simulink model "LC62_PIDControl_V6"  (R2022b)
settings: Solver=ode4  StartTime=0.0  StopTime=SimTime  FixedStep=1/500  RelTol=1e-3
model workspace (MAT data in the model file):
  Tr = 0.1
  freq = 0.002
  hover_w = 0.55
values from neighbouring files (symbols this model uses):
  b = 1.1    [initfun.m]
  c = 0.551    [initfun.m]
  Cll_beta = -0.0518    [initfun.m]
  Cll_del_A = -0.0369 * 5    (= -0.1845)    [initfun.m]
  Cll_del_R = 0.0026    [initfun.m]
  Cll_p = -0.4624    [initfun.m]
  Cll_r = 0.0218    [initfun.m]
  Cm_del_A = 0.001156    [initfun.m]
  Cm_del_E = -0.676    [initfun.m]
  Cn_beta = 0.0866    [initfun.m]
  Cn_del_A = -0.000385    [initfun.m]
  Cn_del_R = -0.0190    (= -0.019)    [initfun.m]
  Cn_p = -0.0048    [initfun.m]
  Cn_r = -0.0723    [initfun.m]
  Cy_beta = -1.1269    [initfun.m]
  Cy_del_R = 0.0534    [initfun.m]
  Cy_p = 0.0    (= 0)    [initfun.m]
  Cy_r = 0.2374    [initfun.m]
  d = 0.849    [initfun.m]
  dx1 = 0.9325+0.049    (= 0.9815)    [initfun.m]
  dx2 = 0.0725-0.049    (= 0.0235)    [initfun.m]
  dx3 = 1.1725-0.049    (= 1.1235)    [initfun.m]
  dy1 = 0.717 + temp_y    (= 0.717)    [initfun.m]
  dy2 = 0.717 - temp_y    (= 0.717)    [initfun.m]
  g = 9.81    [initfun.m]
  m = 41.97    [initfun.m]
  S = S1 + S2    (= 0.8522)    [initfun.m]
  S2 = 0.5898    [initfun.m]
undefined symbols (not defined in the file or in its folder): d2r, Earth, F, Light, MIL, sigbuilder_block, WGS84
libraries: simulink_extras x50, slpidlib x14, simulink x11, dspstat3 x5, aerolibwind2 x3, sharedTrackingLibrary x2, aerolibasang x2, aerolibtransform2 x2, robotcorelib x1, uavutilslib x1, uavalgslib x1, aerolibnav x1
(part 1 of 4)
settings Model: Creator=CNU_UASG  LastModifiedBy=박범준
settings DebuggingCC: UnconnectedInputMsg=warning  UnconnectedOutputMsg=warning  UnconnectedLineMsg=warning  UnderSpecifiedDimensionMsg=warning
settings ModelReferenceCC: EnableRefExpFcnMdlSchedulingChecks=on
settings RTWCC: DLArmComputeVersion=19.05

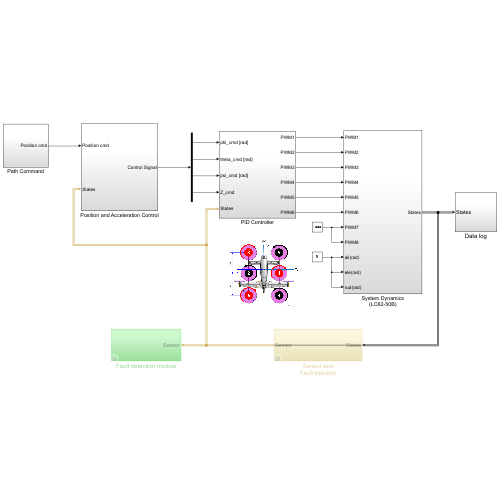
[thumbnail: Simulink's stored preview of the top-level diagram]
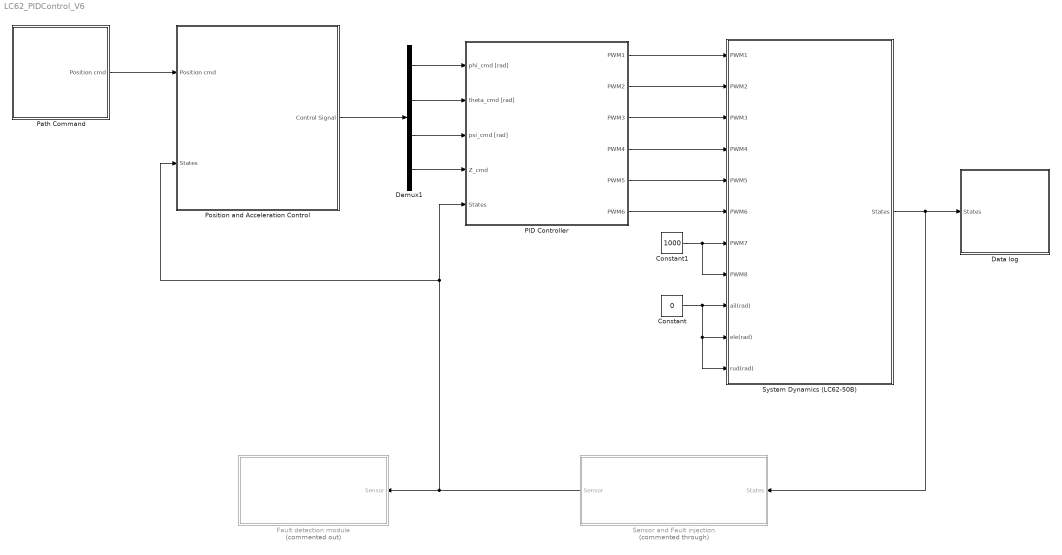
== system LC62_PIDControl_V6 ==
  Constant : Constant  Value=0
  Constant1 : Constant  Value=1000
  Data log : Subsystem
  Demux1 : Demux
  Fault detection module : Subsystem  Commented=on
  PID Controller : Subsystem
  Path Command : Subsystem
  Position and Acceleration Control : Subsystem
  Sensor and Fault injection : Subsystem  Commented=through
  System Dynamics (LC62-50B) : Subsystem
  wires:
  PID Controller/1(PWM1) -> System Dynamics (LC62-50B)/1(PWM1)
  PID Controller/2(PWM2) -> System Dynamics (LC62-50B)/2(PWM2)
  PID Controller/3(PWM3) -> System Dynamics (LC62-50B)/3(PWM3)
  PID Controller/4(PWM4) -> System Dynamics (LC62-50B)/4(PWM4)
  PID Controller/5(PWM5) -> System Dynamics (LC62-50B)/5(PWM5)
  PID Controller/6(PWM6) -> System Dynamics (LC62-50B)/6(PWM6)
  Constant1/1 -> System Dynamics (LC62-50B)/8(PWM8), System Dynamics (LC62-50B)/7(PWM7)
  Constant/1 -> System Dynamics (LC62-50B)/9(ail(rad)), System Dynamics (LC62-50B)/11(rud(rad)), System Dynamics (LC62-50B)/10(ele(rad))
  Demux1/2 -> PID Controller/2(theta_cmd [rad])
  Demux1/1 -> PID Controller/1(phi_cmd [rad])
  Demux1/3 -> PID Controller/3(psi_cmd [rad])
  Demux1/4 -> PID Controller/4(Z_cmd)
  System Dynamics (LC62-50B)/1(States) -> Sensor and Fault injection/1(States), Data log/1(States)
  Position and Acceleration Control/1(Control Signal) -> Demux1/1
  Path Command/1(Position cmd) -> Position and Acceleration Control/1(Position cmd)
  Sensor and Fault injection/1(Sensor) -> Fault detection module/1(Sensor), Position and Acceleration Control/2(States), PID Controller/5(States)

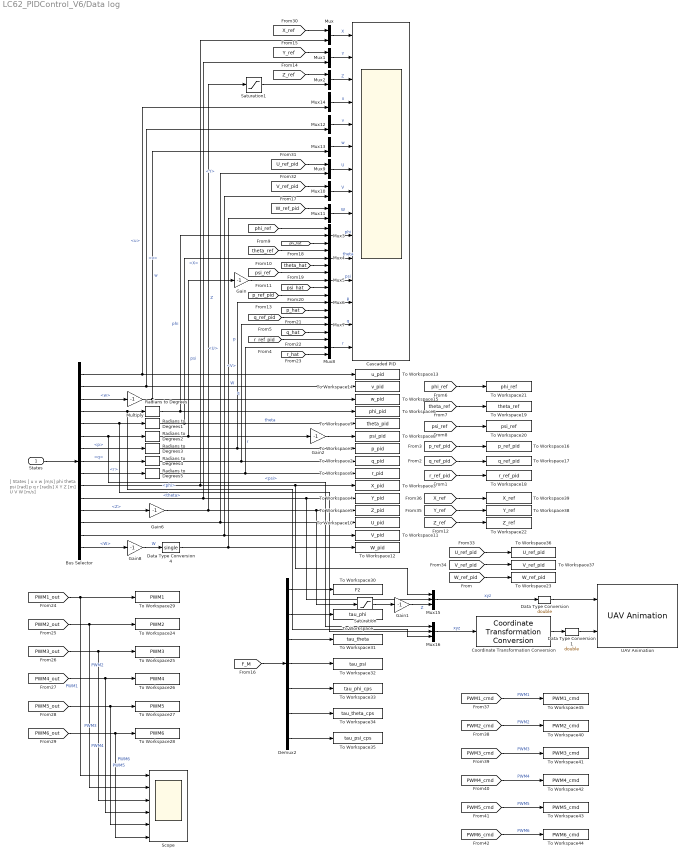
== system LC62_PIDControl_V6/Data log ==
  note: [ States ]
      | u v w [m/s]
      | phi theta psi [rad]
      | p q r [rad/s]
      | X Y Z [m]
      | U V W [m/s]
  States : Inport
  Bus Selector : BusSelector  OutputSignals=u,v,w,phi,theta,psi,p,q,r,X,Y,Z,U,V,W
  Cascaded PID : Scope  NumInputPorts=15
  Coordinate Transformation Conversion : robotcorelib/Coordinate Transformation Conversion  InputRepresentation=Euler Angles  InputEulerSequence=ZYX  ShowTrVecInputPort=on  OutputRepresentation=Quaternion  OutputEulerSequence=ZYX  ShowTrVecOutputPort=on  SimulateUsing=Code generation
  Data Type Conversion : DataTypeConversion  OutDataTypeStr=double  SaturateOnIntegerOverflow=off  RndMeth=Floor
  Data Type Conversion1 : DataTypeConversion  OutDataTypeStr=double  SaturateOnIntegerOverflow=off  RndMeth=Floor
  Data Type Conversion4 : DataTypeConversion  OutDataTypeStr=single  SaturateOnIntegerOverflow=off  RndMeth=Floor
  Demux2 : Demux  Outputs=7
  Gain{,1..2,6,8} (5 alike) : Gain  Gain=-1
  Multiply : Gain  Gain=-1
  Mux{,1..2,9..14} (9 alike) : Mux  Inputs=2
  Mux{3..8,15..16} (8 alike) : Mux  Inputs=3
  Radians to Degrees{,1..5} (6 alike) : simulink_extras/Transformations/Radians to Degrees
  Saturation : Saturate  UpperLimit=500  LowerLimit=0
  Saturation1 : Saturate  UpperLimit=500  LowerLimit=0
  Scope : Scope  NumInputPorts=6
  To Workspace : ToWorkspace  VariableName=tau_phi  SampleTime=-1
  To Workspace1 : ToWorkspace  VariableName=p_pid  SampleTime=-1
  To Workspace10 : ToWorkspace  VariableName=U_pid  SampleTime=-1
  To Workspace11 : ToWorkspace  VariableName=V_pid  SampleTime=-1
  To Workspace12 : ToWorkspace  VariableName=W_pid  SampleTime=-1
  To Workspace13 : ToWorkspace  VariableName=u_pid  SampleTime=-1
  To Workspace14 : ToWorkspace  VariableName=v_pid  SampleTime=-1
  To Workspace15 : ToWorkspace  VariableName=w_pid  SampleTime=-1
  To Workspace16 : ToWorkspace  VariableName=p_ref_pid  SampleTime=-1
  To Workspace17 : ToWorkspace  VariableName=q_ref_pid  SampleTime=-1
  To Workspace18 : ToWorkspace  VariableName=r_ref_pid  SampleTime=-1
  To Workspace19 : ToWorkspace  VariableName=theta_ref  SampleTime=-1
  To Workspace2 : ToWorkspace  VariableName=q_pid  SampleTime=-1
  To Workspace20 : ToWorkspace  VariableName=psi_ref  SampleTime=-1
  To Workspace21 : ToWorkspace  VariableName=phi_ref  SampleTime=-1
  To Workspace22 : ToWorkspace  VariableName=Z_ref  SampleTime=-1
  To Workspace23 : ToWorkspace  VariableName=W_ref_pid  SampleTime=-1
  To Workspace24 : ToWorkspace  VariableName=PWM2  SampleTime=-1
  To Workspace25 : ToWorkspace  VariableName=PWM3  SampleTime=-1
  To Workspace26 : ToWorkspace  VariableName=PWM4  SampleTime=-1
  To Workspace27 : ToWorkspace  VariableName=PWM5  SampleTime=-1
  To Workspace28 : ToWorkspace  VariableName=PWM6  SampleTime=-1
  To Workspace29 : ToWorkspace  VariableName=PWM1  SampleTime=-1
  To Workspace3 : ToWorkspace  VariableName=X_pid  SampleTime=-1
  To Workspace30 : ToWorkspace  VariableName=Fz  SampleTime=-1
  To Workspace31 : ToWorkspace  VariableName=tau_theta  SampleTime=-1
  To Workspace32 : ToWorkspace  VariableName=tau_psi  SampleTime=-1
  To Workspace33 : ToWorkspace  VariableName=tau_phi_cps  SampleTime=-1
  To Workspace34 : ToWorkspace  VariableName=tau_theta_cps  SampleTime=-1
  To Workspace35 : ToWorkspace  VariableName=tau_psi_cps  SampleTime=-1
  To Workspace36 : ToWorkspace  VariableName=U_ref_pid  SampleTime=-1
  To Workspace37 : ToWorkspace  VariableName=V_ref_pid  SampleTime=-1
  To Workspace38 : ToWorkspace  VariableName=Y_ref  SampleTime=-1
  To Workspace39 : ToWorkspace  VariableName=X_ref  SampleTime=-1
  To Workspace4 : ToWorkspace  VariableName=Y_pid  SampleTime=-1
  To Workspace40 : ToWorkspace  VariableName=PWM2_cmd  SampleTime=-1
  To Workspace41 : ToWorkspace  VariableName=PWM3_cmd  SampleTime=-1
  To Workspace42 : ToWorkspace  VariableName=PWM4_cmd  SampleTime=-1
  To Workspace43 : ToWorkspace  VariableName=PWM5_cmd  SampleTime=-1
  To Workspace44 : ToWorkspace  VariableName=PWM6_cmd  SampleTime=-1
  To Workspace45 : ToWorkspace  VariableName=PWM1_cmd  SampleTime=-1
  To Workspace5 : ToWorkspace  VariableName=Z_pid  SampleTime=-1
  To Workspace6 : ToWorkspace  VariableName=phi_pid  SampleTime=-1
  To Workspace7 : ToWorkspace  VariableName=theta_pid  SampleTime=-1
  To Workspace8 : ToWorkspace  VariableName=psi_pid  SampleTime=-1
  To Workspace9 : ToWorkspace  VariableName=r_pid  SampleTime=-1
  UAV Animation : uavutilslib/UAV Animation  UAVType=Multirotor  UAVSize=1  InertialZDirection=Down  SampleTime=1
  wires:
  Bus Selector/12 -> Gain6/1  "<Z>"
  Bus Selector/8 -> Radians to Degrees4/1  "<q>"
  Bus Selector/9 -> Radians to Degrees5/1  "<r>"
  Bus Selector/4 -> Mux16/3, Radians to Degrees/1  "<phi>"
  Bus Selector/5 -> Mux16/2, Radians to Degrees1/1  "<theta>"
  Bus Selector/7 -> Radians to Degrees3/1  "<p>"
  States/1 -> Bus Selector/1
  Bus Selector/15 -> Gain8/1  "<W>"
  Bus Selector/6 -> Mux16/1, Radians to Degrees2/1  "<psi>"
  Bus Selector/3 -> Multiply/1  "<w>"
  Bus Selector/10 -> Mux15/1, To Workspace3/1, Mux/2  "<X>"
  Bus Selector/11 -> Mux15/2, To Workspace4/1, Mux1/2  "<Y>"
  Gain6/1 -> Saturation/1, To Workspace5/1, Saturation1/1  "Z"
  Radians to Degrees3/1 -> To Workspace1/1, Mux6/2  "p"
  Radians to Degrees4/1 -> To Workspace2/1, Mux7/2  "q"
  Radians to Degrees5/1 -> To Workspace9/1, Mux8/2  "r"
  Gain8/1 -> Data Type Conversion4/1  "W"
  Bus Selector/14 -> To Workspace11/1, Mux10/2  "<V>"
  Bus Selector/13 -> To Workspace10/1, Mux9/2  "<U>"
  Radians to Degrees2/1 -> Gain2/1, Gain/1  "psi"
  Radians to Degrees1/1 -> To Workspace7/1, Mux4/2  "theta"
  Radians to Degrees/1 -> To Workspace6/1, Mux3/2  "phi"
  Multiply/1 -> To Workspace15/1, Mux13/2  "w"
  Bus Selector/2 -> To Workspace14/1, Mux12/2  "<v>"
  Bus Selector/1 -> Mux14/2, To Workspace13/1  "<u>"
  Mux2/1 -> Cascaded PID/3  "Z"
  Mux/1 -> Cascaded PID/1  "X"
  Mux1/1 -> Cascaded PID/2  "Y"
  Mux10/1 -> Cascaded PID/8  "V"
  Mux9/1 -> Cascaded PID/7  "U"
  Mux11/1 -> Cascaded PID/9  "W"
  Mux13/1 -> Cascaded PID/6  "w"
  Mux12/1 -> Cascaded PID/5  "v"
  [q_ref_pid] -> Mux7/1
  [p_ref_pid] -> Mux6/1
  [r_ref_pid] -> Mux8/1
  Mux3/1 -> Cascaded PID/10  "phi"
  Mux4/1 -> Cascaded PID/11  "theta"
  Mux5/1 -> Cascaded PID/12  "psi"
  Mux6/1 -> Cascaded PID/13  "p"
  Mux7/1 -> Cascaded PID/14  "q"
  Mux8/1 -> Cascaded PID/15  "r"
  [psi_ref] -> To Workspace20/1
  [phi_ref] -> To Workspace21/1
  [theta_ref] -> To Workspace19/1
  [phi_ref] -> Mux3/1
  [theta_ref] -> Mux4/1
  [psi_ref] -> Mux5/1
  [Z_ref] -> To Workspace22/1
  [Z_ref] -> Mux2/1
  [W_ref_pid] -> To Workspace23/1
  [p_ref_pid] -> To Workspace16/1
  [q_ref_pid] -> To Workspace17/1
  [r_ref_pid] -> To Workspace18/1
  [F_M] -> Demux2/1
  Demux2/5 -> To Workspace33/1
  Demux2/6 -> To Workspace34/1
  Demux2/7 -> To Workspace35/1
  Demux2/4 -> To Workspace32/1
  Demux2/3 -> To Workspace31/1
  Demux2/2 -> To Workspace/1
  Demux2/1 -> To Workspace30/1
  [W_ref_pid] -> Mux11/1
  [PWM1_out] -> Scope/1, To Workspace29/1  "PWM1"
  [PWM2_out] -> Scope/2, To Workspace24/1  "PWM2"
  [PWM3_out] -> Scope/3, To Workspace25/1  "PWM3"
  [PWM4_out] -> Scope/4, To Workspace26/1  "PWM4"
  [PWM5_out] -> Scope/5, To Workspace27/1  "PWM5"
  [PWM6_out] -> To Workspace28/1, Scope/6  "PWM6"
  [phi_hat] -> Mux3/3
  [theta_hat] -> Mux4/3
  [psi_hat] -> Mux5/3
  [p_hat] -> Mux6/3
  [q_hat] -> Mux7/3
  [r_hat] -> Mux8/3
  Coordinate Transformation Conversion/1 -> Data Type Conversion1/1
  Data Type Conversion/1 -> UAV Animation/1
  Mux15/1 -> Data Type Conversion/1  "xyz"
  Mux16/1 -> Coordinate Transformation Conversion/1  "xyz"
  Data Type Conversion4/1 -> To Workspace12/1, Mux11/2  "W"
  [Y_ref] -> Mux1/1
  [X_ref] -> Mux/1
  Data Type Conversion1/1 -> UAV Animation/2
  Gain1/1 -> Mux15/3  "Z"
  [U_ref_pid] -> Mux9/1
  [V_ref_pid] -> Mux10/1
  Mux14/1 -> Cascaded PID/4  "u"
  [U_ref_pid] -> To Workspace36/1
  [V_ref_pid] -> To Workspace37/1
  [Y_ref] -> To Workspace38/1
  [X_ref] -> To Workspace39/1
  [PWM6_cmd] -> To Workspace44/1  "PWM6"
  [PWM5_cmd] -> To Workspace43/1  "PWM5"
  [PWM4_cmd] -> To Workspace42/1  "PWM4"
  [PWM3_cmd] -> To Workspace41/1  "PWM3"
  [PWM2_cmd] -> To Workspace40/1  "PWM2"
  [PWM1_cmd] -> To Workspace45/1  "PWM1"
  Saturation/1 -> Gain1/1
  Saturation1/1 -> Mux2/2
  Gain/1 -> Mux5/2
  Gain2/1 -> To Workspace8/1

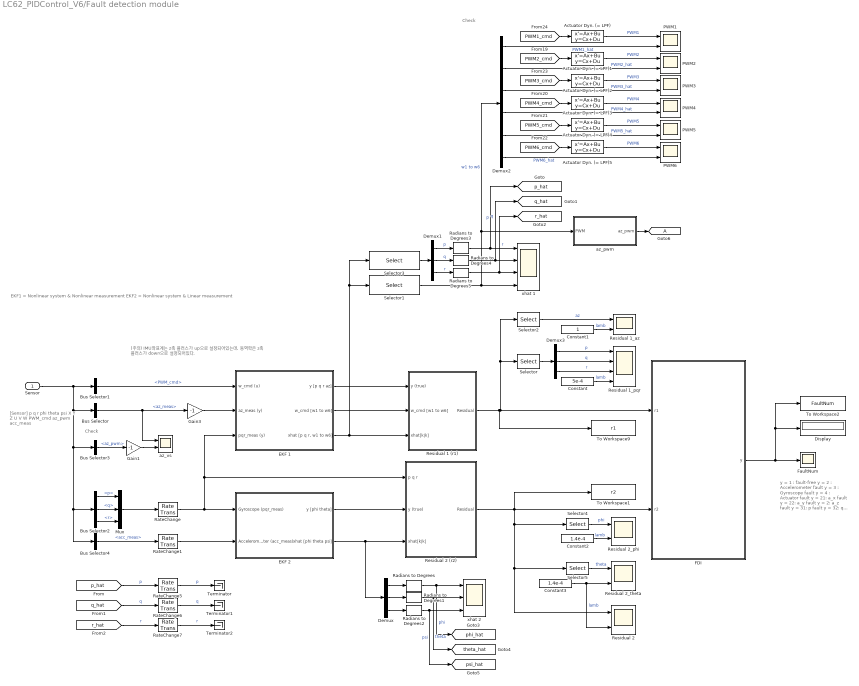
== system LC62_PIDControl_V6/Fault detection module ==
  note: (주의) IMU좌표계는 z축 플러스가 up으로 설정되어있는데,
      | 동역학은 z축 플러스가 down으로 설정되어있다.
  note: Check
  note: y = 1 : fault-free
      | y = 2 : Accelerometer fault
      | y = 3 : Gyroscope fault
      | y = 4 : Actuator fault
      |
      | y = 21: a_x fault
      | y = 22: a_y fault
      | y = 2: a_z fault
      |
      | y = 31: p fault
      | y = 32: q fault
      | y = 33: r fault
  note: EKF1 = Nonlinear system & Nonlinear measurement
      |
      | EKF2 = Nonlinear system & Linear measurement
  note: [Sensor]
      | p q r
      | phi theta psi
      | X Y Z
      | U V W
      | PWM_cmd
      | az_pwm
      | acc_meas
  note: Check
  Sensor : Inport
  Actuator Dyn. (= LPF){,1..5} (6 alike) : StateSpace  A=-1/Tr  B=1/Tr  D=0  InitialCondition=hover_w
  Bus Selector : BusSelector  OutputSignals=acc_meas.az_meas
  Bus Selector1 : BusSelector  OutputSignals=PWM_cmd
  Bus Selector2 : BusSelector  OutputSignals=p,q,r
  Bus Selector3 : BusSelector  OutputSignals=az_pwm
  Bus Selector4 : BusSelector  OutputSignals=acc_meas
  Constant : Constant  Value=5e-4
  Constant1 : Constant
  Constant2 : Constant  Value=1.4e-4
  Constant3 : Constant  Value=1.4e-4
  Demux : Demux  Outputs=3
  Demux1 : Demux  Outputs=3
  Demux2 : Demux  Outputs=6
  Demux3 : Demux  Outputs=3
  Display : Display
  EKF 1 : Subsystem
  EKF 2 : Subsystem
  FDI : MATLAB Function  TreatAsAtomicUnit=on
  FaultNum : Scope
  Gain1 : Gain  Gain=-1
  Gain3 : Gain  Gain=-1
  Goto6 : Goto  TagVisibility=global
  Mux : Mux  Inputs=3
  PWM{1..6} (6 alike) : Scope  NumInputPorts=2
  Radians to Degrees{,1..5} (6 alike) : simulink_extras/Transformations/Radians to Degrees
  RateChange : RateTransition  OutPortSampleTime=0.05
  RateChange1 : RateTransition  OutPortSampleTime=0.05
  RateChange5 : RateTransition  OutPortSampleTime=1/500
  RateChange6 : RateTransition  OutPortSampleTime=1/500
  RateChange7 : RateTransition  OutPortSampleTime=1/500
  Residual 1 (r1) : Subsystem
  Residual 1_az : Scope  NumInputPorts=2
  Residual 1_pqr : Scope  NumInputPorts=4
  Residual 2 : Scope  NumInputPorts=2
  Residual 2 (r2) : Subsystem
  Residual 2_phi : Scope  NumInputPorts=2
  Residual 2_theta : Scope  NumInputPorts=2
  Selector : Selector  InputPortWidth=4  IndexOptions=Index vector (dialog)  Indices=[1:3]  OutputSizes=1
  Selector1 : Selector  InputPortWidth=9  IndexOptions=Index vector (dialog)  Indices=[4:9]  OutputSizes=1
  Selector2 : Selector  InputPortWidth=4  IndexOptions=Index vector (dialog)  Indices=[4]  OutputSizes=1
  Selector3 : Selector  InputPortWidth=9  IndexOptions=Index vector (dialog)  Indices=[1:3]  OutputSizes=1
  Selector4 : Selector  InputPortWidth=2  IndexOptions=Index vector (dialog)  Indices=[1]  OutputSizes=1
  Selector5 : Selector  InputPortWidth=2  IndexOptions=Index vector (dialog)  Indices=[2]  OutputSizes=1
  Terminator : Terminator
  Terminator1 : Terminator
  Terminator2 : Terminator
  To Workspace1 : ToWorkspace  VariableName=r2  SampleTime=-1
  To Workspace2 : ToWorkspace  VariableName=FaultNum  SampleTime=-1
  To Workspace9 : ToWorkspace  VariableName=r1  SampleTime=-1
  az_pwm : MATLAB Function  TreatAsAtomicUnit=on
  az_vs : Scope  NumInputPorts=2
  xhat 1 : Scope  NumInputPorts=4
  xhat 2 : Scope  NumInputPorts=3
  tag scope: p_hat=global, phi_hat=global, psi_hat=global, q_hat=global, r_hat=global, theta_hat=global
  wires:
  Sensor/1 -> Bus Selector/1, Bus Selector3/1, Bus Selector4/1, Bus Selector2/1, Bus Selector1/1
  [q_hat] -> RateChange6/1  "q"
  Demux1/2 -> Radians to Degrees4/1  "q"
  EKF 1/2(w_cmd [w1 to w6]) -> Residual 1 (r1)/2(w_cmd [w1 to w6])
  Selector4/1 -> Residual 2_phi/1  "phi"
  Radians to Degrees2/1 -> xhat 2/3, [psi_hat]  "psi"
  Radians to Degrees5/1 -> [r_hat], xhat 1/3  "r"
  EKF 1/3("xhat [p q r, w1 to w6]") -> Residual 1 (r1)/3(xhat[k|k]), Selector3/1, Selector1/1
  EKF 1/1(y [p q r az]) -> Residual 1 (r1)/1(y (true))
  RateChange5/1 -> Terminator/1  "p"
  Demux1/3 -> Radians to Degrees5/1  "r"
  Demux/1 -> Radians to Degrees/1
  Radians to Degrees/1 -> xhat 2/1, [phi_hat]  "phi"
  EKF 2/1(y [phi theta]) -> Residual 2 (r2)/2(y (true))
  Radians to Degrees1/1 -> xhat 2/2, [theta_hat]  "theta"
  Gain3/1 -> EKF 1/2(az_meas (y))
  Bus Selector2/3 -> Mux/3  "<r>"
  Bus Selector4/1 -> RateChange1/1  "<acc_meas>"
  Bus Selector2/1 -> Mux/1  "<p>"
  FDI/1(y) -> To Workspace2/1, Display/1, FaultNum/1
  Demux1/1 -> Radians to Degrees3/1  "p"
  RateChange6/1 -> Terminator1/1  "q"
  Selector1/1 -> Demux2/1, az_pwm/1(PWM), xhat 1/4  "w1 to w6"
  Bus Selector/1 -> Gain3/1, az_vs/1  "<az_meas>"
  Selector3/1 -> Demux1/1
  [r_hat] -> RateChange7/1  "r"
  [p_hat] -> RateChange5/1  "p"
  EKF 2/2(xhat [phi theta psi]) -> Demux/1, Residual 2 (r2)/3(xhat[k|k])
  RateChange1/1 -> EKF 2/2(Accelerometer (acc_meas))
  Bus Selector2/2 -> Mux/2  "<q>"
  Bus Selector1/1 -> EKF 1/1(w_cmd (u))  "<PWM_cmd>"
  RateChange7/1 -> Terminator2/1  "r"
  Residual 1 (r1)/1(Residual) -> Selector/1, Selector2/1, FDI/1(r1), To Workspace9/1
  RateChange/1 -> Residual 2 (r2)/1(p q r), EKF 1/3(pqr_meas (y)), EKF 2/1(Gyroscope (pqr_meas))
  Demux/2 -> Radians to Degrees1/1
  Radians to Degrees3/1 -> [p_hat], xhat 1/1  "p"
  Residual 2 (r2)/1(Residual) -> Selector5/1, Residual 2/1, Selector4/1, FDI/2(r2), To Workspace1/1
  Mux/1 -> RateChange/1
  Radians to Degrees4/1 -> [q_hat], xhat 1/2  "q"
  Demux/3 -> Radians to Degrees2/1
  Bus Selector3/1 -> Gain1/1  "<az_pwm>"
  [PWM1_cmd] -> Actuator Dyn. (= LPF)/1
  [PWM2_cmd] -> Actuator Dyn. (= LPF)1/1
  [PWM3_cmd] -> Actuator Dyn. (= LPF)2/1
  [PWM4_cmd] -> Actuator Dyn. (= LPF)3/1
  [PWM5_cmd] -> Actuator Dyn. (= LPF)4/1
  [PWM6_cmd] -> Actuator Dyn. (= LPF)5/1
  Gain1/1 -> az_vs/2
  Demux3/1 -> Residual 1_pqr/1  "p"
  Demux3/2 -> Residual 1_pqr/2  "q"
  Demux3/3 -> Residual 1_pqr/3  "r"
  Selector/1 -> Demux3/1
  Constant/1 -> Residual 1_pqr/4  "lamb"
  Selector2/1 -> Residual 1_az/1  "az"
  Constant1/1 -> Residual 1_az/2  "lamb"
  Actuator Dyn. (= LPF)/1 -> PWM1/1  "PWM1"
  Actuator Dyn. (= LPF)1/1 -> PWM2/1  "PWM2"
  Actuator Dyn. (= LPF)2/1 -> PWM3/1  "PWM3"
  Actuator Dyn. (= LPF)3/1 -> PWM4/1  "PWM4"
  Actuator Dyn. (= LPF)4/1 -> PWM5/1  "PWM5"
  Actuator Dyn. (= LPF)5/1 -> PWM6/1  "PWM6"
  Demux2/1 -> PWM1/2  "PWM1_hat"
  Demux2/2 -> PWM2/2  "PWM2_hat"
  Demux2/3 -> PWM3/2  "PWM3_hat"
  Demux2/4 -> PWM4/2  "PWM4_hat"
  Demux2/5 -> PWM5/2  "PWM5_hat"
  Demux2/6 -> PWM6/2  "PWM6_hat"
  Constant2/1 -> Residual 2_phi/2  "lamb"
  Selector5/1 -> Residual 2_theta/1  "theta"
  Constant3/1 -> Residual 2/2, Residual 2_theta/2  "lamb"
  az_pwm/1(az_pwm) -> Goto6/1

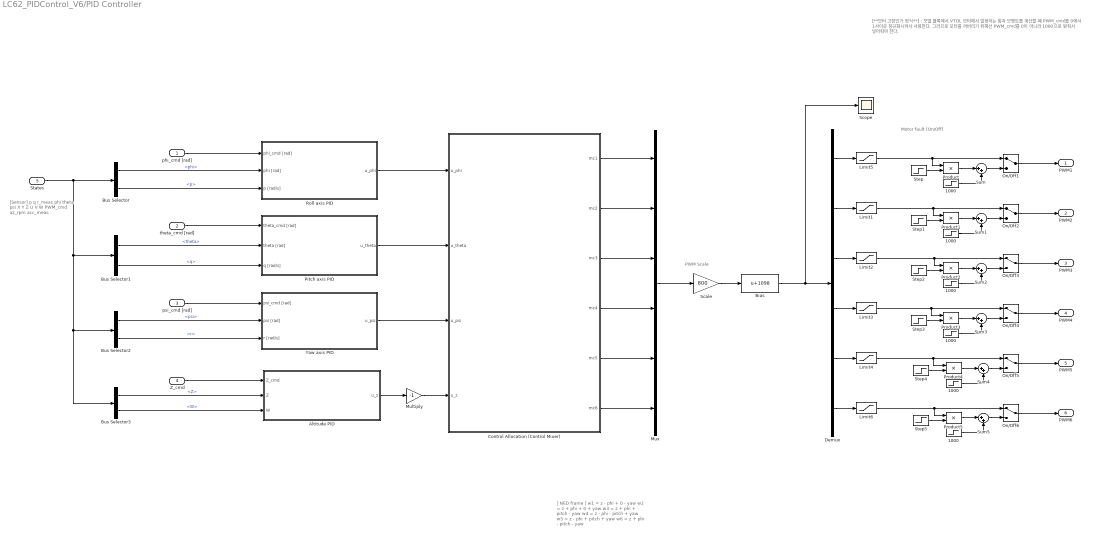
== system LC62_PIDControl_V6/PID Controller ==
  note: [**모터 고장인가 방식**]
      |
      | : 모델 블록에서 VTOL 모터에서 발생하는 힘과 모멘트를 계산할 때 PWM_cmd를 0에서 1사이로 정규화시켜서 사용한다. 그러므로 모터를 꺼버리기 위해선 PWM_cmd를 0이 아니라 1000으로 맞춰서 넣어줘야 한다.
  note: [Sensor]
      | p q r_meas
      | phi theta psi
      | X Y Z
      | U V W
      | PWM_cmd
      | az_rpm
      | acc_meas
  note: PWM Scale
  note: [ NED frame ]
      |
      | w1 = z - phi + 0 - yaw
      |
      | w2 = z + phi + 0 + yaw
      |
      | w3 = z + phi + pitch - yaw
      |
      | w4 = z - phi - pitch + yaw
      |
      | w5 = z - phi + pitch + yaw
      |
      | w6 = z + phi - pitch - yaw
  note: Motor fault (On/Off)
  phi_cmd [rad] : Inport
  theta_cmd [rad] : Inport  Port=2
  psi_cmd [rad] : Inport  Port=3
  Z_cmd : Inport  Port=4
  States : Inport  Port=5
  "   1000   " : Step  Time=5  After=1000
  "  1000  " : Step  Time=5  After=1000
  " 1000 " : Step  Time=5  After=1000
  " 1000  " : Step  Time=5  After=1000
  1000 : Step  Time=5  After=1000
  "1000 " : Step  Time=5  After=1000
  Altitude PID : Subsystem
  Bias : Bias  Bias=1098  SaturateOnIntegerOverflow=off
  Bus Selector : BusSelector  OutputSignals=phi,p
  Bus Selector1 : BusSelector  OutputSignals=theta,q
  Bus Selector2 : BusSelector  OutputSignals=psi,r
  Bus Selector3 : BusSelector  OutputSignals=Z,W
  Control Allocation (Control Mixer) : MATLAB Function  TreatAsAtomicUnit=on
  Demux : Demux  Outputs=6
  Limit{1..6} (6 alike) : Saturate  UpperLimit=2000  LowerLimit=1000
      settings: AttributesFormatString=%<LowerLimit>~%<UpperLimit>
  Multiply : Gain  Gain=-1
  Mux : Mux  Inputs=6
  On/Off{1..6} (6 alike) : ManualSwitch
  Pitch axis PID : Subsystem
  Product{,1..5} (6 alike) : Product
  Roll axis PID : Subsystem
  Scale : Gain  Gain=800
  Scope : Scope
  Step{,1..5} (6 alike) : Step  Time=5  Before=1  After=0
  Sum{,1..5} (6 alike) : Sum  Inputs=|++
  Yaw axis PID : Subsystem
  PWM1 : Outport
  PWM2 : Outport  Port=2
  PWM3 : Outport  Port=3
  PWM4 : Outport  Port=4
  PWM5 : Outport  Port=5
  PWM6 : Outport  Port=6
  wires:
  psi_cmd [rad]/1 -> Yaw axis PID/1(psi_cmd [rad])
  Pitch axis PID/1(u_theta) -> Control Allocation (Control Mixer)/2(u_theta)
  Z_cmd/1 -> Altitude PID/1(Z_cmd)
  Roll axis PID/1(u_phi) -> Control Allocation (Control Mixer)/1(u_phi)
  Yaw axis PID/1(u_psi) -> Control Allocation (Control Mixer)/3(u_psi)
  Control Allocation (Control Mixer)/4(mc4) -> Mux/4
  Bias/1 -> Demux/1, Scope/1
  Multiply/1 -> Control Allocation (Control Mixer)/4(u_z)
  Mux/1 -> Scale/1
  Control Allocation (Control Mixer)/1(mc1) -> Mux/1
  Demux/6 -> Limit6/1
  Control Allocation (Control Mixer)/6(mc6) -> Mux/6
  Demux/1 -> Limit5/1
  States/1 -> Bus Selector/1, Bus Selector2/1, Bus Selector3/1, Bus Selector1/1
  Scale/1 -> Bias/1
  phi_cmd [rad]/1 -> Roll axis PID/1(phi_cmd [rad])
  Demux/2 -> Limit1/1
  Demux/4 -> Limit3/1
  Bus Selector/2 -> Roll axis PID/3(p [rad/s])  "<p>"
  Bus Selector3/1 -> Altitude PID/2(Z)  "<Z>"
  Control Allocation (Control Mixer)/3(mc3) -> Mux/3
  Altitude PID/1(u_z) -> Multiply/1
  Bus Selector3/2 -> Altitude PID/3(W)  "<W>"
  theta_cmd [rad]/1 -> Pitch axis PID/1(theta_cmd [rad])
  Bus Selector2/2 -> Yaw axis PID/3(r [rad/s])  "<r>"
  Bus Selector1/1 -> Pitch axis PID/2(theta [rad])  "<theta>"
  Bus Selector1/2 -> Pitch axis PID/3(q [rad/s])  "<q>"
  Control Allocation (Control Mixer)/5(mc5) -> Mux/5
  Demux/3 -> Limit2/1
  Bus Selector/1 -> Roll axis PID/2(phi [rad])  "<phi>"
  Demux/5 -> Limit4/1
  Bus Selector2/1 -> Yaw axis PID/2(psi [rad])  "<psi>"
  Control Allocation (Control Mixer)/2(mc2) -> Mux/2
  Limit5/1 -> On/Off1/1, Product/1
  On/Off1/1 -> PWM1/1
  On/Off2/1 -> PWM2/1
  Limit1/1 -> Product1/1, On/Off2/1
  Limit2/1 -> Product2/1, On/Off3/1
  On/Off3/1 -> PWM3/1
  Limit3/1 -> Product3/1, On/Off4/1
  On/Off4/1 -> PWM4/1
  Limit4/1 -> Product4/1, On/Off5/1
  On/Off5/1 -> PWM5/1
  Limit6/1 -> Product5/1, On/Off6/1
  On/Off6/1 -> PWM6/1
  Product/1 -> Sum/1
  1000/1 -> Sum/2
  Sum/1 -> On/Off1/2
  Step/1 -> Product/2
  "1000 "/1 -> Sum1/2
  Product1/1 -> Sum1/1
  Step1/1 -> Product1/2
  Sum1/1 -> On/Off2/2
  Product2/1 -> Sum2/1
  Step2/1 -> Product2/2
  " 1000  "/1 -> Sum2/2
  Sum2/1 -> On/Off3/2
  Step3/1 -> Product3/2
  "   1000   "/1 -> Sum3/2
  Product3/1 -> Sum3/1
  Sum3/1 -> On/Off4/2
  Step4/1 -> Product4/2
  "  1000  "/1 -> Sum4/2
  Product4/1 -> Sum4/1
  Sum4/1 -> On/Off5/2
  Product5/1 -> Sum5/1
  Step5/1 -> Product5/2
  " 1000 "/1 -> Sum5/2
  Sum5/1 -> On/Off6/2

== system LC62_PIDControl_V6/Path Command ==
  Constant : Constant  Value=0
  Constant1 : Constant  Commented=on  Value=[0 0 150; 20 20 150; -20 20 150; -20 -20 150; 20 -20 150; 20 20 150; 0 0 150]  VectorParams1D=off
  Constant3 : Constant  Commented=on  Value=[0 0 150 0.25*pi; 20 20 150 pi; -20 20 150 -0.5*pi; -20 -20 150 0; 20 -20 150 0.5*pi; 20 20 150 0.5*pi; 0 0 150 0.25*pi]  VectorParams1D=off
  Constant5 : Constant  Commented=on  Value=40
  Data Type Conversion{1..4} (4 alike) : DataTypeConversion  OutDataTypeStr=single  SaturateOnIntegerOverflow=off  RndMeth=Floor
  From1 : From  Commented=on  GotoTag=Pose_PID
  Gain : Gain  Gain=-1
  Gain2 : Gain  Gain=1/2
  Gain3 : Gain  Gain=1/2
  Gain4 : Gain  Gain=1/5
  Manual Switch : ManualSwitch  CurrentSetting=0
  Manual Switch1 : ManualSwitch  CurrentSetting=0
  Manual Switch2 : ManualSwitch  CurrentSetting=0
  Manual Switch3 : ManualSwitch
  Mux1 : Mux
  Reshape : Reshape  Commented=on  OutputDimensionality=Column vector (2-D)
  Signal Builder1 : Subsystem  Tag=STV Subsys  Commented=on  LoadFcn=sigbuilder_block('load');  StartFcn=sigbuilder_block('start');  StopFcn=sigbuilder_block('stop');  ClipboardFcn=sigbuilder_block('clipboard');  mask(Sigbuilder block){tuvar=[0:10]}
      mask help: Simulink:masks:SigbuilderBlock_MD
      mask init:
      | if ~strcmp(get_param(bdroot(gcbh),'SimulationStatus'),'stopped') tuvar = sigbuilder_block('maskInit'); end
      settings: CopyFcn=sigbuilder_block('copy');  DeleteFcn=sigbuilder_block('delete');  ModelCloseFcn=sigbuilder_block('modelClose');  PreSaveFcn=sigbuilder_block('preSave');  PauseFcn=sigbuilder_block('pause');  ContinueFcn=sigbuilder_block('continue');  NameChangeFcn=sigbuilder_block('namechange');  OpenFcn=sigbuilder_block('open',[-1289.25 383.25 1137.75 338.25 ]);  CloseFcn=sigbuilder_block('close');
      mask Display: plot(0, 0, 100, 100,[2, 2, 32, 32, 2], [68, 8, 8, 68, 68],[32, 2], [38, 38], [32, 19, 2],[53, 60, 44], [32, 17, 17, 2],[16, 16, 31, 31]);txt = getActiveGroup(gcbh);text(2, 100, txt,'verticalAlignment', 'top');
  Signal Builder2 : Subsystem  Tag=STV Subsys  Commented=on  LoadFcn=sigbuilder_block('load');  StartFcn=sigbuilder_block('start');  StopFcn=sigbuilder_block('stop');  ClipboardFcn=sigbuilder_block('clipboard');  mask(Sigbuilder block){tuvar=[0:10]}
      mask help: Simulink:masks:SigbuilderBlock_MD
      mask init:
      | if ~strcmp(get_param(bdroot(gcbh),'SimulationStatus'),'stopped') tuvar = sigbuilder_block('maskInit'); end
      settings: CopyFcn=sigbuilder_block('copy');  DeleteFcn=sigbuilder_block('delete');  ModelCloseFcn=sigbuilder_block('modelClose');  PreSaveFcn=sigbuilder_block('preSave');  PauseFcn=sigbuilder_block('pause');  ContinueFcn=sigbuilder_block('continue');  NameChangeFcn=sigbuilder_block('namechange');  OpenFcn=sigbuilder_block('open',[-1296 45.75 1137.75 353.25 ]);  CloseFcn=sigbuilder_block('close');
      mask Display: plot(0, 0, 100, 100,[2, 2, 32, 32, 2], [68, 8, 8, 68, 68],[32, 2], [38, 38], [32, 19, 2],[53, 60, 44], [32, 17, 17, 2],[16, 16, 31, 31]);txt = getActiveGroup(gcbh);text(2, 100, txt,'verticalAlignment', 'top');
  Signal Builder3 : Subsystem  Tag=STV Subsys  Commented=on  LoadFcn=sigbuilder_block('load');  StartFcn=sigbuilder_block('start');  StopFcn=sigbuilder_block('stop');  ClipboardFcn=sigbuilder_block('clipboard');  mask(Sigbuilder block){tuvar=[0:10]}
      mask help: Simulink:masks:SigbuilderBlock_MD
      mask init:
      | if ~strcmp(get_param(bdroot(gcbh),'SimulationStatus'),'stopped') tuvar = sigbuilder_block('maskInit'); end
      settings: CopyFcn=sigbuilder_block('copy');  DeleteFcn=sigbuilder_block('delete');  ModelCloseFcn=sigbuilder_block('modelClose');  PreSaveFcn=sigbuilder_block('preSave');  PauseFcn=sigbuilder_block('pause');  ContinueFcn=sigbuilder_block('continue');  NameChangeFcn=sigbuilder_block('namechange');  OpenFcn=sigbuilder_block('open',[296.25 222 1137.75 338.25 ]);  CloseFcn=sigbuilder_block('close');
      mask Display: plot(0, 0, 100, 100,[2, 2, 32, 32, 2], [68, 8, 8, 68, 68],[32, 2], [38, 38], [32, 19, 2],[53, 60, 44], [32, 17, 17, 2],[16, 16, 31, 31]);txt = getActiveGroup(gcbh);text(2, 100, txt,'verticalAlignment', 'top');
  Signal Builder4 : Subsystem  Tag=STV Subsys  Commented=on  LoadFcn=sigbuilder_block('load');  StartFcn=sigbuilder_block('start');  StopFcn=sigbuilder_block('stop');  ClipboardFcn=sigbuilder_block('clipboard');  mask(Sigbuilder block){tuvar=[0:10]}
      mask help: Simulink:masks:SigbuilderBlock_MD
      mask init:
      | if ~strcmp(get_param(bdroot(gcbh),'SimulationStatus'),'stopped') tuvar = sigbuilder_block('maskInit'); end
      settings: CopyFcn=sigbuilder_block('copy');  DeleteFcn=sigbuilder_block('delete');  ModelCloseFcn=sigbuilder_block('modelClose');  PreSaveFcn=sigbuilder_block('preSave');  PauseFcn=sigbuilder_block('pause');  ContinueFcn=sigbuilder_block('continue');  NameChangeFcn=sigbuilder_block('namechange');  OpenFcn=sigbuilder_block('open',[296.25 222 1137.75 338.25 ]);  CloseFcn=sigbuilder_block('close');
      mask Display: plot(0, 0, 100, 100,[2, 2, 32, 32, 2], [68, 8, 8, 68, 68],[32, 2], [38, 38], [32, 19, 2],[53, 60, 44], [32, 17, 17, 2],[16, 16, 31, 31]);txt = getActiveGroup(gcbh);text(2, 100, txt,'verticalAlignment', 'top');
  Transfer Fcn1 : TransferFcn  Commented=through  Denominator=[3 1]
  Transfer Fcn2 : TransferFcn  Commented=through  Denominator=[3 1]
  Transfer Fcn3 : TransferFcn  Commented=through  Denominator=[3 1]
  Waypoint Command (원점 기준 +-20m 간격 사각경로) : Subsystem  Tag=STV Subsys  LoadFcn=sigbuilder_block('load');  StartFcn=sigbuilder_block('start');  StopFcn=sigbuilder_block('stop');  ClipboardFcn=sigbuilder_block('clipboard');  mask(Sigbuilder block){tuvar=[0:10]}
      mask help: Simulink:masks:SigbuilderBlock_MD
      mask init:
      | if ~strcmp(get_param(bdroot(gcbh),'SimulationStatus'),'stopped') tuvar = sigbuilder_block('maskInit'); end
      settings: CopyFcn=sigbuilder_block('copy');  DeleteFcn=sigbuilder_block('delete');  ModelCloseFcn=sigbuilder_block('modelClose');  PreSaveFcn=sigbuilder_block('preSave');  PauseFcn=sigbuilder_block('pause');  ContinueFcn=sigbuilder_block('continue');  NameChangeFcn=sigbuilder_block('namechange');  OpenFcn=sigbuilder_block('open',[183.75 138.75 1141.5 444.75 ]);  CloseFcn=sigbuilder_block('close');
      mask Display: plot(0, 0, 100, 100,[2, 2, 32, 32, 2], [68, 8, 8, 68, 68],[32, 2], [38, 38], [32, 19, 2],[53, 60, 44], [32, 17, 17, 2],[16, 16, 31, 31]);txt = getActiveGroup(gcbh);text(2, 100, txt,'verticalAlignment', 'top');
  Waypoint Follower1 : uavalgslib/Waypoint Follower  Commented=on  UAVType=multirotor  StartFrom=first  TransitionRadiusSource=internal  TransitionRadius=20  MinLookaheadDistance=0.1  YawInput=off  ShowCrossTrackErrorOutput=off  ShowStatusOutput=off  SimulateUsing=Interpreted execution
  Position cmd : Outport
  tag scope: X_ref=global, Y_ref=global, Z_ref=global
  wires:
  Mux1/1 -> Position cmd/1
  Data Type Conversion4/1 -> Mux1/1, [X_ref]
  Data Type Conversion1/1 -> Mux1/2, [Y_ref]
  Data Type Conversion2/1 -> Gain/1, [Z_ref]
  Data Type Conversion3/1 -> Mux1/4
  Gain/1 -> Mux1/3
  Manual Switch/1 -> Data Type Conversion4/1  "[m]"
  Waypoint Command (원점 기준 +-20m 간격 사각경로)/3(Z_cmd) -> Gain4/1
  Manual Switch1/1 -> Data Type Conversion1/1  "[m]"
  Manual Switch2/1 -> Data Type Conversion2/1  "[m]"
  Transfer Fcn3/1 -> Manual Switch2/2
  Gain3/1 -> Transfer Fcn1/1
  Gain4/1 -> Transfer Fcn3/1
  Waypoint Command (원점 기준 +-20m 간격 사각경로)/2(Y_cmd) -> Gain3/1
  Transfer Fcn1/1 -> Manual Switch1/2
  Reshape/1 -> Waypoint Follower1/1
  Gain2/1 -> Transfer Fcn2/1
  Waypoint Command (원점 기준 +-20m 간격 사각경로)/1(X_cmd) -> Gain2/1
  Transfer Fcn2/1 -> Manual Switch/2
  Manual Switch3/1 -> Data Type Conversion3/1  "[rad]"
  Constant/1 -> Manual Switch2/1, Manual Switch3/1, Manual Switch1/1, Manual Switch/1
  Constant5/1 -> Waypoint Follower1/3
  Waypoint Follower1/2 -> Manual Switch3/2
  Constant1/1 -> Waypoint Follower1/2
  From1/1 -> Reshape/1

== system LC62_PIDControl_V6/Position and Acceleration Control ==
  Position cmd : Inport
  States : Inport  Port=2
  Acceleration Control : Subsystem
  Data Type Conversion4 : DataTypeConversion  OutDataTypeStr=single  SaturateOnIntegerOverflow=off  RndMeth=Floor
  Position Control : Subsystem
  Velocity Control : Subsystem
  Control Signal : Outport
  wires:
  Position cmd/1 -> Data Type Conversion4/1, Position Control/1(Position cmd)
  States/1 -> Velocity Control/2(States), Acceleration Control/2(States), Position Control/2(States)
  Position Control/1(Velocity Cmd) -> Velocity Control/1(Velocity Cmd)
  Acceleration Control/1(Control Signal) -> Control Signal/1
  Velocity Control/1(Accel Cmd) -> Acceleration Control/1(Accel Cmd)
  Data Type Conversion4/1 -> Acceleration Control/3(Position cmd)

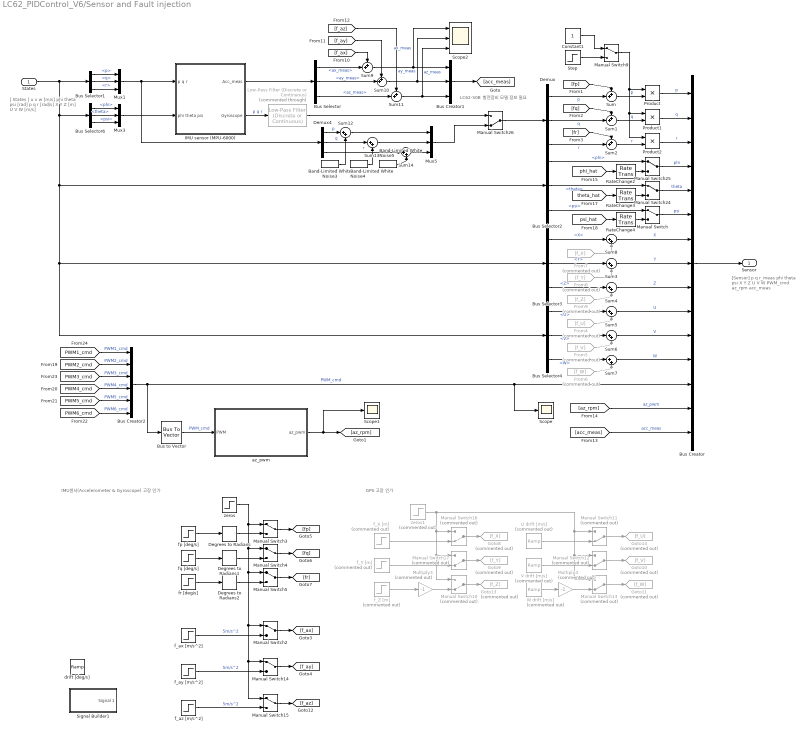
== system LC62_PIDControl_V6/Sensor and Fault injection ==
  note: IMU센서(Accelerometer & Gyroscope) 고장 인가
  note: GPS 고장 인가
  note: [Sensor]
      | p q r_meas
      | phi theta psi
      | X Y Z
      | U V W
      | PWM_cmd
      | az_rpm
      | acc_meas
  note: [ States ]
      | u v w [m/s]
      | phi theta psi [rad]
      | p q r [rad/s]
      | X Y Z [m]
      | U V W [m/s]
  note: LC62-50B 항전장비 모델 정보 필요
  States : Inport
  Band-Limited White Noise3 : simulink/Sources/Band-Limited White Noise  Cov=[5e-10]  Ts=1/freq  seed=[189621]
  Band-Limited White Noise4 : simulink/Sources/Band-Limited White Noise  Cov=[5e-10]  Ts=1/freq  seed=[128794]
  Band-Limited White Noise5 : simulink/Sources/Band-Limited White Noise  Cov=[5e-10]  Ts=1/freq  seed=[214632]
  Bus Creator : BusCreator  Inputs=15
  Bus Creator1 : BusCreator  Inputs=3
  Bus Creator2 : BusCreator  Inputs=6
  Bus Selector : BusSelector  OutputSignals=ax_meas,ay_meas,az_meas
  Bus Selector1 : BusSelector  OutputSignals=p,q,r
  Bus Selector2 : BusSelector  OutputSignals=phi,theta,psi
  Bus Selector3 : BusSelector  OutputSignals=X,Y,Z
  Bus Selector4 : BusSelector  OutputSignals=U,V,W
  Bus Selector6 : BusSelector  OutputSignals=phi,theta,psi
  Bus to Vector : BusToVector
  Constant1 : Constant
  Degrees to Radians : simulink_extras/Transformations/Degrees to Radians
  Degrees to Radians1 : simulink_extras/Transformations/Degrees to Radians
  Degrees to Radians2 : simulink_extras/Transformations/Degrees to Radians
  Demux : Demux  Outputs=3
  Demux4 : Demux  Outputs=3
  From4 : From  Commented=on  GotoTag=f_U  TagVisibility=global
  From5 : From  Commented=on  GotoTag=f_V  TagVisibility=global
  From6 : From  Commented=on  GotoTag=f_W  TagVisibility=global
  From7 : From  Commented=on  GotoTag=f_X  TagVisibility=global
  From8 : From  Commented=on  GotoTag=f_Y  TagVisibility=global
  From9 : From  Commented=on  GotoTag=f_Z  TagVisibility=global
  Goto10 : Goto  Commented=on  GotoTag=f_V
  Goto11 : Goto  Commented=on  GotoTag=f_W
  Goto13 : Goto  Commented=on  GotoTag=f_Z
  Goto14 : Goto  Commented=on  GotoTag=f_U
  Goto8 : Goto  Commented=on  GotoTag=f_X
  Goto9 : Goto  Commented=on  GotoTag=f_Y
  IMU sensor (MPU-6000) : Subsystem
  Low-Pass Filter (Discrete or Continuous) : eeGeneralControl/Low-Pass Filter (Discrete or Continuous)  Commented=through  K=1  T=0.02  B=inf  A=-inf  init_option=Inherited from block input  x0=0  Ts=-1
  Manual Switch{,2..5,9,14..15,24..25} (10 alike) : ManualSwitch
  Manual Switch{10..13,16..17} (6 alike) : ManualSwitch  Commented=on  CurrentSetting=0
  Manual Switch26 : ManualSwitch  CurrentSetting=0
  Multiply3 : Gain  Commented=on  Gain=-1
  Multiply4 : Gain  Commented=on  Gain=-1
  Mux1 : Mux  Inputs=3
  Mux3 : Mux  Inputs=3
  Mux5 : Mux  Inputs=3
  Product : Product
  Product1 : Product
  Product2 : Product
  RateChange2 : RateTransition  OutPortSampleTime=1/500
  RateChange3 : RateTransition  OutPortSampleTime=1/500
  RateChange4 : RateTransition  OutPortSampleTime=1/500
  Scope : Scope
  Scope1 : Scope
  Scope2 : Scope  NumInputPorts=3
  Signal Builder1 : Subsystem  Tag=STV Subsys  LoadFcn=sigbuilder_block('load');  StartFcn=sigbuilder_block('start');  StopFcn=sigbuilder_block('stop');  ClipboardFcn=sigbuilder_block('clipboard');  mask(Sigbuilder block){tuvar=[0:10]}
      mask help: Simulink:masks:SigbuilderBlock_MD
      mask init:
      | if ~strcmp(get_param(bdroot(gcbh),'SimulationStatus'),'stopped') tuvar = sigbuilder_block('maskInit'); end
      settings: CopyFcn=sigbuilder_block('copy');  DeleteFcn=sigbuilder_block('delete');  ModelCloseFcn=sigbuilder_block('modelClose');  PreSaveFcn=sigbuilder_block('preSave');  PauseFcn=sigbuilder_block('pause');  ContinueFcn=sigbuilder_block('continue');  NameChangeFcn=sigbuilder_block('namechange');  OpenFcn=sigbuilder_block('open',[311.25 180 724.5 439.5 ]);  CloseFcn=sigbuilder_block('close');
      mask Display: plot(0, 0, 100, 100,[2, 2, 32, 32, 2], [68, 8, 8, 68, 68],[32, 2], [38, 38], [32, 19, 2],[53, 60, 44], [32, 17, 17, 2],[16, 16, 31, 31]);txt = getActiveGroup(gcbh);text(2, 100, txt,'verticalAlignment', 'top');
  Step : Step  Time=5  Before=1  After=0.5
  Sum{,1..2,9..11} (6 alike) : Sum  Inputs=++|
  Sum{3..8,12..14} (9 alike) : Sum  Inputs=|++
  U drift [m/s] : simulink/Sources/Ramp  Commented=on  slope=0.01  start=5  InitialOutput=0
  V drift [m/s] : simulink/Sources/Ramp  Commented=on  slope=0.01  start=5  InitialOutput=0
  W drift [m/s] : simulink/Sources/Ramp  Commented=on  slope=0.01  start=5  InitialOutput=0
  az_pwm : MATLAB Function  TreatAsAtomicUnit=on
  drift [deg/s] : simulink/Sources/Ramp  slope=1  start=5  InitialOutput=0
  f_X [m] : Step  Commented=on  Time=0  After=10  SampleTime=0
  f_Y [m] : Step  Commented=on  Time=0  After=10  SampleTime=0
  f_Z [m] : Step  Commented=on  Time=0  After=5  SampleTime=0
  f_ax [m/s^2] : Step  Time=5  After=5
  f_ay [m/s^2] : Step  Time=5  After=5
  f_az [m/s^2] : Step  Time=5  After=5
  fp [deg/s] : Step  Time=5  After=5  SampleTime=0
  fq [deg/s] : Step  Time=5  After=5  SampleTime=0
  fr [deg/s] : Step  Time=5  After=5  SampleTime=0
  zeros : Step  Time=0  After=0  SampleTime=0
  zeros1 : Step  Commented=on  Time=0  After=0  SampleTime=0
  Sensor : Outport
  wires:
  IMU sensor (MPU-6000)/1(Acc_meas) -> Bus Selector/1
  IMU sensor (MPU-6000)/2(Gyroscope) -> Low-Pass Filter (Discrete or Continuous)/1  "p q r"
  Demux/2 -> Sum1/2  "q"
  Demux/1 -> Sum/2  "p"
  Demux/3 -> Sum2/2  "r"
  [fp] -> Sum/1
  [fq] -> Sum1/1
  [fr] -> Sum2/1
  Bus Selector4/1 -> Sum5/1  "<U>"
  Sum5/1 -> Bus Creator/10  "U"
  Bus Selector4/2 -> Sum6/1  "<V>"
  Sum6/1 -> Bus Creator/11  "V"
  Bus Selector4/3 -> Sum7/1  "<W>"
  Sum7/1 -> Bus Creator/12  "W"
  Sum3/1 -> Bus Creator/8  "Y"
  Bus Selector3/2 -> Sum3/1  "<Y>"
  Sum4/1 -> Bus Creator/9  "Z"
  Bus Selector3/3 -> Sum4/1  "<Z>"
  f_ay [m/s^2]/1 -> Manual Switch14/2  "5m/s^2"
  f_az [m/s^2]/1 -> Manual Switch15/2  "5m/s^2"
  Manual Switch2/1 -> [f_ax]
  Manual Switch15/1 -> [f_az]
  Manual Switch3/1 -> [fp]
  f_ax [m/s^2]/1 -> Manual Switch2/2  "5m/s^2"
  Manual Switch5/1 -> [fr]
  Degrees to Radians1/1 -> Manual Switch4/2
  fp [deg/s]/1 -> Degrees to Radians/1
  Manual Switch4/1 -> [fq]
  Degrees to Radians/1 -> Manual Switch3/2
  zeros/1 -> Manual Switch4/1, Manual Switch15/1, Manual Switch14/1, Manual Switch2/1, Manual Switch5/1, Manual Switch3/1
  fq [deg/s]/1 -> Degrees to Radians1/1
  fr [deg/s]/1 -> Degrees to Radians2/1
  Degrees to Radians2/1 -> Manual Switch5/2
  Manual Switch14/1 -> [f_ay]
  Bus Selector/2 -> Sum10/2  "<ay_meas>"
  Bus Selector/3 -> Sum11/2  "<az_meas>"
  Sum10/1 -> Scope2/2, Bus Creator1/2  "ay_meas"
  Sum11/1 -> Scope2/3, Bus Creator1/3  "az_meas"
  Sum9/1 -> Scope2/1, Bus Creator1/1  "ax_meas"
  Bus Creator1/1 -> [acc_meas]
  Product/1 -> Bus Creator/1  "p"
  Sum/1 -> Product/2  "p"
  Product1/1 -> Bus Creator/2  "q"
  Sum1/1 -> Product1/2  "q"
  Product2/1 -> Bus Creator/3  "r"
  Sum2/1 -> Product2/2  "r"
  Constant1/1 -> Manual Switch9/1
  Manual Switch9/1 -> Product/1, Product2/1, Product1/1
  Step/1 -> Manual Switch9/2
  Manual Switch12/1 -> Goto10/1
  Manual Switch10/1 -> Goto13/1
  Manual Switch13/1 -> Goto11/1
  f_X [m]/1 -> Manual Switch16/2
  Manual Switch16/1 -> Goto8/1
  Manual Switch11/1 -> Goto14/1
  U drift [m/s]/1 -> Manual Switch11/2
  V drift [m/s]/1 -> Manual Switch12/2
  Multiply4/1 -> Manual Switch13/2
  f_Y [m]/1 -> Manual Switch17/2
  W drift [m/s]/1 -> Multiply4/1
  zeros1/1 -> Manual Switch12/1, Manual Switch13/1, Manual Switch11/1, Manual Switch16/1, Manual Switch17/1, Manual Switch10/1
  f_Z [m]/1 -> Multiply3/1
  Multiply3/1 -> Manual Switch10/2
  Manual Switch17/1 -> Goto9/1
  [acc_meas] -> Bus Creator/15  "acc_meas"
  Manual Switch25/1 -> Bus Creator/4  "phi"
  Manual Switch24/1 -> Bus Creator/5  "theta"
  Manual Switch/1 -> Bus Creator/6  "psi"
  [phi_hat] -> RateChange2/1
  RateChange2/1 -> Manual Switch25/2
  Bus Selector2/1 -> Manual Switch25/1  "<phi>"
  Bus Selector2/2 -> Manual Switch24/1  "<theta>"
  Bus Selector2/3 -> Manual Switch/1  "<psi>"
  [theta_hat] -> RateChange3/1
  RateChange3/1 -> Manual Switch24/2
  [psi_hat] -> RateChange4/1
  RateChange4/1 -> Manual Switch/2
  Bus Selector3/1 -> Sum8/1  "<X>"
  Sum8/1 -> Bus Creator/7  "X"
  From7/1 -> Sum8/2
  From8/1 -> Sum3/2
  From9/1 -> Sum4/2
  From4/1 -> Sum5/2
  From5/1 -> Sum6/2
  From6/1 -> Sum7/2
  Bus Selector1/1 -> Mux1/1  "<p>"
  Bus Selector1/2 -> Mux1/2  "<q>"
  Bus Selector1/3 -> Mux1/3  "<r>"
  Mux1/1 -> Demux4/1, IMU sensor (MPU-6000)/1(p q r)
  Mux3/1 -> IMU sensor (MPU-6000)/2(phi theta psi)
  Bus Selector/1 -> Sum9/2  "<ax_meas>"
  [f_ax] -> Sum9/1
  [f_ay] -> Sum10/1
  [f_az] -> Sum11/1
  States/1 -> Bus Selector4/1, Bus Selector3/1, Bus Selector2/1, Bus Selector6/1, Bus Selector1/1
  Bus Creator/1 -> Sensor/1
  [az_rpm] -> Bus Creator/14  "az_pwm"
  Bus Selector6/2 -> Mux3/2  "<theta>"
  Bus Selector6/1 -> Mux3/1  "<phi>"
  Bus Selector6/3 -> Mux3/3  "<psi>"
  Low-Pass Filter (Discrete or Continuous)/1 -> Manual Switch26/1
  Manual Switch26/1 -> Demux/1
  az_pwm/1(az_pwm) -> Scope1/1, [az_rpm]
  Bus to Vector/1 -> az_pwm/1(PWM)  "PWM_cmd"
  [PWM1_cmd] -> Bus Creator2/1  "PWM1_cmd"
  [PWM2_cmd] -> Bus Creator2/2  "PWM2_cmd"
  [PWM3_cmd] -> Bus Creator2/3  "PWM3_cmd"
  [PWM4_cmd] -> Bus Creator2/4  "PWM4_cmd"
  [PWM5_cmd] -> Bus Creator2/5  "PWM5_cmd"
  [PWM6_cmd] -> Bus Creator2/6  "PWM6_cmd"
  Bus Creator2/1 -> Scope/1, Bus Creator/13, Bus to Vector/1  "PWM_cmd"
  Sum12/1 -> Mux5/1
  Band-Limited White Noise3/1 -> Sum12/2
  Demux4/2 -> Sum13/1  "q"
  Demux4/3 -> Sum14/1  "r"
  Band-Limited White Noise5/1 -> Sum14/2
  Sum14/1 -> Mux5/3
  Demux4/1 -> Sum12/1  "p"
  Band-Limited White Noise4/1 -> Sum13/2
  Sum13/1 -> Mux5/2
  Mux5/1 -> Manual Switch26/2

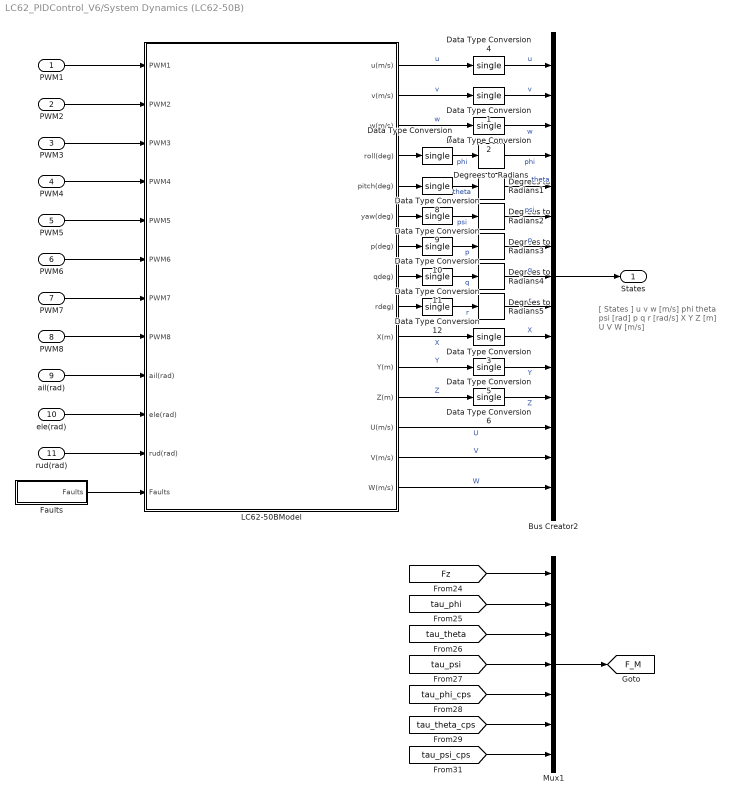
== system LC62_PIDControl_V6/System Dynamics (LC62-50B) ==
  note: [ States ]
      | u v w [m/s]
      | phi theta psi [rad]
      | p q r [rad/s]
      | X Y Z [m]
      | U V W [m/s]
  PWM1 : Inport
  PWM2 : Inport  Port=2
  PWM3 : Inport  Port=3
  PWM4 : Inport  Port=4
  PWM5 : Inport  Port=5
  PWM6 : Inport  Port=6
  PWM7 : Inport  Port=7
  PWM8 : Inport  Port=8
  ail(rad) : Inport  Port=9
  ele(rad) : Inport  Port=10
  rud(rad) : Inport  Port=11
  Bus Creator2 : BusCreator  Inputs=15
  Data Type Conversion{1..12} (12 alike) : DataTypeConversion  OutDataTypeStr=single  SaturateOnIntegerOverflow=off  RndMeth=Floor
  Degrees to Radians{,1..5} (6 alike) : simulink_extras/Transformations/Degrees to Radians
  Faults : Subsystem
  LC62-50BModel : Subsystem
  Mux1 : Mux  Inputs=7
  States : Outport
  tag scope: F_M=global
  wires:
  Bus Creator2/1 -> States/1
  LC62-50BModel/11(Y(m)) -> Data Type Conversion5/1  "Y"
  Degrees to Radians4/1 -> Bus Creator2/8  "q"
  LC62-50BModel/12(Z(m)) -> Data Type Conversion6/1  "Z"
  LC62-50BModel/14(V(m/s)) -> Bus Creator2/14  "V"
  Degrees to Radians3/1 -> Bus Creator2/7  "p"
  LC62-50BModel/15(W(m/s)) -> Bus Creator2/15  "W"
  LC62-50BModel/13(U(m/s)) -> Bus Creator2/13  "U"
  LC62-50BModel/3(w(m/s)) -> Data Type Conversion2/1  "w"
  LC62-50BModel/1(u(m/s)) -> Data Type Conversion4/1  "u"
  Degrees to Radians2/1 -> Bus Creator2/6  "psi"
  PWM1/1 -> LC62-50BModel/1(PWM1)
  PWM4/1 -> LC62-50BModel/4(PWM4)
  LC62-50BModel/4(roll(deg)) -> Data Type Conversion7/1
  PWM8/1 -> LC62-50BModel/8(PWM8)
  LC62-50BModel/2(v(m/s)) -> Data Type Conversion1/1  "v"
  rud(rad)/1 -> LC62-50BModel/11(rud(rad))
  LC62-50BModel/9(rdeg)) -> Data Type Conversion12/1
  PWM6/1 -> LC62-50BModel/6(PWM6)
  PWM7/1 -> LC62-50BModel/7(PWM7)
  [tau_theta] -> Mux1/3
  PWM5/1 -> LC62-50BModel/5(PWM5)
  PWM3/1 -> LC62-50BModel/3(PWM3)
  [tau_psi] -> Mux1/4
  Degrees to Radians5/1 -> Bus Creator2/9  "r"
  [tau_theta_cps] -> Mux1/6
  [tau_phi] -> Mux1/2
  Degrees to Radians1/1 -> Bus Creator2/5  "theta"
  [tau_phi_cps] -> Mux1/5
  LC62-50BModel/10(X(m)) -> Data Type Conversion3/1  "X"
  [Fz] -> Mux1/1
  LC62-50BModel/6(yaw(deg)) -> Data Type Conversion9/1
  Mux1/1 -> [F_M]
  LC62-50BModel/5(pitch(deg)) -> Data Type Conversion8/1
  LC62-50BModel/8(qdeg)) -> Data Type Conversion11/1
  PWM2/1 -> LC62-50BModel/2(PWM2)
  [tau_psi_cps] -> Mux1/7
  ele(rad)/1 -> LC62-50BModel/10(ele(rad))
  ail(rad)/1 -> LC62-50BModel/9(ail(rad))
  Degrees to Radians/1 -> Bus Creator2/4  "phi"
  LC62-50BModel/7(p(deg)) -> Data Type Conversion10/1
  Faults/1(Faults) -> LC62-50BModel/12(Faults)
  Data Type Conversion4/1 -> Bus Creator2/1  "u"
  Data Type Conversion1/1 -> Bus Creator2/2  "v"
  Data Type Conversion2/1 -> Bus Creator2/3  "w"
  Data Type Conversion3/1 -> Bus Creator2/10  "X"
  Data Type Conversion5/1 -> Bus Creator2/11  "Y"
  Data Type Conversion6/1 -> Bus Creator2/12  "Z"
  Data Type Conversion7/1 -> Degrees to Radians/1  "phi"
  Data Type Conversion8/1 -> Degrees to Radians1/1  "theta"
  Data Type Conversion9/1 -> Degrees to Radians2/1  "psi"
  Data Type Conversion10/1 -> Degrees to Radians3/1  "p"
  Data Type Conversion11/1 -> Degrees to Radians4/1  "q"
  Data Type Conversion12/1 -> Degrees to Radians5/1  "r"

== system LC62_PIDControl_V6/Fault detection module/EKF 1 ==
  note: [ EKF1 : Using Dynamics ]
      | x = [p q r, w1, w2, w3, w4, w5, w6]'
      | y = [p q r, az]'
  note: [IMU센서 가속도계 노이즈 값]
      | 0.0000001
  w_cmd (u) : Inport
  az_meas (y) : Inport  Port=2
  pqr_meas (y) : Inport  Port=3
  Band-Limited White Noise : simulink/Sources/Band-Limited White Noise  Cov=[1e-7]  Ts=1/freq  seed=[23341]
  Extended Kalman Filter 1 : sharedTrackingLibrary/Extended Kalman Filter  StateTransitionFcn=EKF1_fn_fx  HasStateTransitionJacobianFcn=on  StateTransitionJacobianFcn=EKF1_fn_JF  HasAdditiveProcessNoise=Additive  ProcessNoise=1e-2*diag(ones(9,1))  HasTimeVaryingProcessNoise=off  HasStateTransitionFcnExtraArgument=1  InitialState=[0;0;0;(0.55)*ones(6,1)]  InitialStateCovariance=1e-4*eye(9)  MeasurementFcn1=EKF1_fn_hx  HasMeasurementJacobianFcn1=on  MeasurementJacobianFcn1=EKF1_fn_JH  HasMeasurementEnablePort1=off  HasAdditiveMeasurementNoise1=Additive  MeasurementNoise1=1e-4*diag(ones(4,1))  HasTimeVaryingMeasurementNoise1=off  HasMeasurementFcnExtraArgument1=0  HasMeasurementWrapping1=off  MeasurementFcn2=myMeasurementFcn  HasMeasurementJacobianFcn2=off  HasMeasurementEnablePort2=off  HasAdditiveMeasurementNoise2=Additive  MeasurementNoise2=1  HasTimeVaryingMeasurementNoise2=off  HasMeasurementFcnExtraArgument2=0  HasMeasurementWrapping2=off  MeasurementFcn3=myMeasurementFcn  HasMeasurementJacobianFcn3=off  HasMeasurementEnablePort3=off  HasAdditiveMeasurementNoise3=Additive  MeasurementNoise3=1  HasTimeVaryingMeasurementNoise3=off  HasMeasurementFcnExtraArgument3=0  HasMeasurementWrapping3=off  MeasurementFcn4=myMeasurementFcn  HasMeasurementJacobianFcn4=off  HasMeasurementEnablePort4=off  HasAdditiveMeasurementNoise4=Additive  MeasurementNoise4=1  HasTimeVaryingMeasurementNoise4=off  HasMeasurementFcnExtraArgument4=0  HasMeasurementWrapping4=off  MeasurementFcn5=myMeasurementFcn  HasMeasurementJacobianFcn5=off  HasMeasurementEnablePort5=off  HasAdditiveMeasurementNoise5=Additive  MeasurementNoise5=1  HasTimeVaryingMeasurementNoise5=off  HasMeasurementFcnExtraArgument5=0  HasMeasurementWrapping5=off  EnableMultirate=off  StateTransitionFcnSampleTime=1  MeasurementFcn1SampleTime=1  MeasurementFcn2SampleTime=1  MeasurementFcn3SampleTime=1  MeasurementFcn4SampleTime=1  MeasurementFcn5SampleTime=1  UseCurrentEstimator=on  OutputStateCovariance=on  DataType=double  SampleTime=0.05  NumberOfMeasurements=1
  Mux2 : Mux  Inputs=2
  RateChange : RateTransition  OutPortSampleTime=0.05
  RateChange1 : RateTransition  OutPortSampleTime=0.05
  Scope : Scope
  Sum : Sum  Inputs=|++
  y [p q r az] : Outport
  w_cmd [w1 to w6] : Outport  Port=2
  "xhat [p q r, w1 to w6]" : Outport  Port=3
  wires:
  Extended Kalman Filter 1/2 -> Scope/1
  w_cmd (u)/1 -> RateChange1/1
  Extended Kalman Filter 1/1 -> "xhat [p q r, w1 to w6]"/1  "[p q r, w1 to w6]"
  pqr_meas (y)/1 -> Mux2/1  "p q r"
  RateChange1/1 -> Extended Kalman Filter 1/1, w_cmd [w1 to w6]/1  "w_cmd"
  Band-Limited White Noise/1 -> Sum/2
  az_meas (y)/1 -> Sum/1
  Mux2/1 -> Extended Kalman Filter 1/2, y [p q r az]/1
  RateChange/1 -> Mux2/2  "az"
  Sum/1 -> RateChange/1
